simulink model "btdonghocbai6"  (R2022b)
settings: Solver=VariableStepAuto  StartTime=0.0  StopTime=10.0  RelTol=1e-3
settings Model: Creator=admin  LastModifiedBy=admin

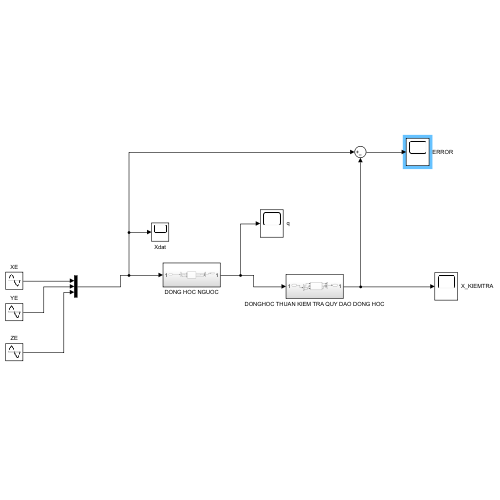
[thumbnail: Simulink's stored preview of the top-level diagram]
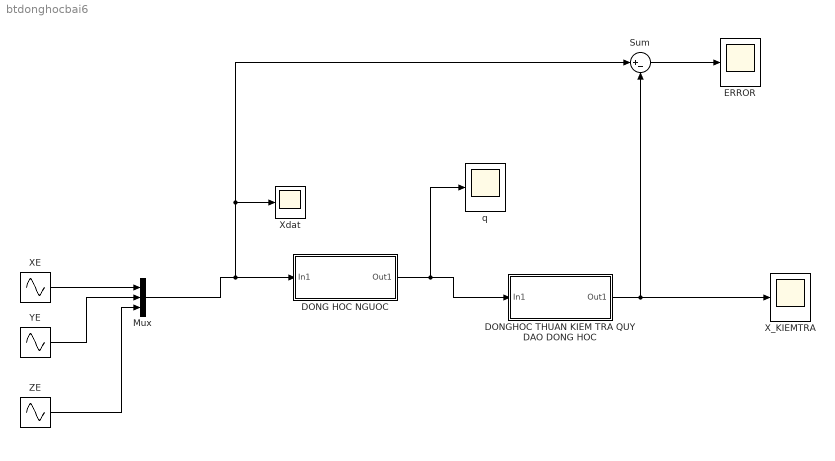
== system btdonghocbai6 ==
  DONG HOC NGUOC : Subsystem
  DONGHOC THUAN KIEM TRA QUY DAO DONG HOC : Subsystem
  ERROR : Scope
  Mux : Mux  Inputs=3
  Sum : Sum  Inputs=|+-
  XE : Sin  Amplitude=0.01  Bias=1  Frequency=0  Phase=-pi/2  SampleTime=0
  X_KIEMTRA : Scope
  Xdat : Scope
  YE : Sin  Amplitude=0.03  Bias=1  SampleTime=0
  ZE : Sin  Amplitude=0.02  Bias=1  Phase=pi/2  SampleTime=0
  q : Scope
  wires:
  XE/1 -> Mux/1
  YE/1 -> Mux/2
  Mux/1 -> Sum/1, Xdat/1, DONG HOC NGUOC/1(In1)
  DONG HOC NGUOC/1(Out1) -> q/1, DONGHOC THUAN KIEM TRA QUY DAO DONG HOC/1(In1)
  DONGHOC THUAN KIEM TRA QUY DAO DONG HOC/1(Out1) -> X_KIEMTRA/1, Sum/2
  Sum/1 -> ERROR/1
  ZE/1 -> Mux/3

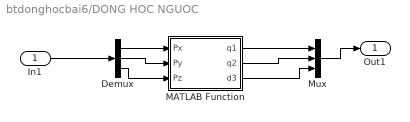
== system btdonghocbai6/DONG HOC NGUOC ==
  In1 : Inport
  Demux : Demux  Outputs=3
  MATLAB Function : MATLAB Function  TreatAsAtomicUnit=on
  Mux : Mux  Inputs=3
  Out1 : Outport
  wires:
  Demux/1 -> MATLAB Function/1(Px)
  Demux/2 -> MATLAB Function/2(Py)
  In1/1 -> Demux/1
  MATLAB Function/1(q1) -> Mux/1
  MATLAB Function/2(q2) -> Mux/2
  Mux/1 -> Out1/1
  Demux/3 -> MATLAB Function/3(Pz)
  MATLAB Function/3(d3) -> Mux/3

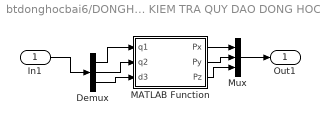
== system btdonghocbai6/DONGHOC THUAN KIEM TRA QUY DAO DONG HOC ==
  In1 : Inport
  Demux : Demux  Outputs=3
  MATLAB Function : MATLAB Function  TreatAsAtomicUnit=on
  Mux : Mux  Inputs=3
  Out1 : Outport
  wires:
  In1/1 -> Demux/1
  Demux/1 -> MATLAB Function/1(q1)
  Demux/2 -> MATLAB Function/2(q2)
  MATLAB Function/1(Px) -> Mux/1
  MATLAB Function/2(Py) -> Mux/2
  Mux/1 -> Out1/1
  Demux/3 -> MATLAB Function/3(d3)
  MATLAB Function/3(Pz) -> Mux/3

== matlab function btdonghocbai6/DONGHOC THUAN KIEM TRA QUY DAO DONG HOC/MATLAB Function ==
  data: Px output; q1 input; Py output; q2 input; d3 input; Pz output
function [Px, Py, Pz] = fcn(q1,q2,d3)
d2=1;
Px = cos(q1)*sin(q2)*d3-sin(q1)*d2;
Py = sin(q1)*sin(q2)*d3+cos(q1)*d2;
Pz = cos(q2)*d3;
end

== matlab function btdonghocbai6/DONG HOC NGUOC/MATLAB Function ==
  data: Px input; q1 output; Py input; q2 output; Pz input; d3 output
function [q1, q2, d3] = fcn(Px, Py, Pz)
d2 = 1;
t = (-Px+sqrt(abs(Px^2+Py^2-d2^2)))/(d2+Py);
c1 = (1-t^2)/(1+t^2);
s1 = 2*t/(1+t^2);
q1 = 2*atan2(-Px+sqrt(abs(Px^2+Py^2-d2^2)),d2+Py);
q2 = atan2((Px*c1+Py*s1),Pz);
d3 = sqrt(abs((Px*c1+Py*s1)^2+Pz^2));
end
